simulink library "exampleMicrogridLibrary"  (R2020a)
settings: Solver=VariableStepAuto  StartTime=0.0  StopTime=10.0  RelTol=1e-3
undefined symbols (not defined in the file): BR, D1, Delta, DiscIntNeverNeededParam, Fnom, gcbh, Ion, kv, Lithium, Ls, Rs, sps_rtmsupport, StationData, Ts, Ts_Control, Vrms
libraries: powerlib x75, simulink x29, powerlib_meascontrol x26, sps_avr x5, spsDieselMotorModel x3, electricdrivelib x2, re_lib x1
(part 6 of 6)

== system exampleMicrogridLibrary/Grid-Connected Battery (Multi-mode EMT Model)/Inverter Control/Current Control/Current Regulator ==
  note: Current Regulator
      | ================
  note: Sign Convention: Current going out of the converter = positive current
  note: Iq positive --> The converter absorbs reactive power ("Inductive mode") = Reactive Power Q negative
  note: Id positive --> The converter generates active power ("Inverter mode") = Active Power P positive
  VdVq_meas : Inport  PortDimensions=2
  IdIq_meas : Inport  Port=2  PortDimensions=2
  IdIq_ref : Inport  Port=3  PortDimensions=2
  Add1 : Sum  Inputs=++-
  Add2 : Sum
  Add3 : Sum  Inputs=+++
  Demux : Demux  Outputs=2
  Demux1 : Demux  Outputs=2
  Lff : Gain  Gain=Ltot_pu  SaturateOnIntegerOverflow=on  OutDataTypeStr=Inherit: Same as input  ParamDataTypeStr=Inherit: Same as input
  "Lff  " : Gain  Gain=Ltot_pu  SaturateOnIntegerOverflow=on  OutDataTypeStr=Inherit: Same as input  ParamDataTypeStr=Inherit: Same as input
  Mux : Mux  Inputs=2
  PI : simulink/Continuous/PID Controller  Controller=PI  Form=Parallel  TimeDomain=Discrete-time  UseExternalTs=off  SampleTime=Ts_Control  IntegratorMethod=Forward Euler  FilterMethod=Forward Euler  ControllerParametersSource=internal  P=Kp_Ireg  I=Ki_Ireg  D=0  UseFilter=on  N=100  TunerSelectOption=Transfer Function Based (PID Tuner App)  InitialConditionSource=internal  InitialConditionForIntegrator=0  InitialConditionForFilter=0  DifferentiatorICPrevScaledInput=0  ExternalReset=none  TrackingMode=off  Kt=1  LimitOutput=on  UpperSaturationLimit=1.5  LowerSaturationLimit=-1.5  LinearizeAsGain=off  AntiWindupMode=clamping  Kb=1  POutMin=[]  POutMax=[]  IOutMin=[]  IOutMax=[]  DOutMin=[]  DOutMax=[]  NOutMin=[]  NOutMax=[]  SumOutMin=[]  SumOutMax=[]  SaturationOutMin=[]  SaturationOutMax=[]  PParamMin=[]  PParamMax=[]  IParamMin=[]  IParamMax=[]  DParamMin=[]  DParamMax=[]  NParamMin=[]  NParamMax=[]  KbParamMin=[]  KbParamMax=[]  KtParamMin=[]  KtParamMax=[]  KbOutMin=[]  KbOutMax=[]  KtOutMin=[]  KtOutMax=[]  IntegratorOutMin=[]  IntegratorOutMax=[]  FilterOutMin=[]  FilterOutMax=[]  SumI1OutMin=[]  SumI1OutMax=[]  SumI2OutMin=[]  SumI2OutMax=[]  SumI3OutMin=[]  SumI3OutMax=[]  SumI4OutMin=[]  SumI4OutMax=[]  SumDOutMin=[]  SumDOutMax=[]  DifferentiatorOutMin=[]  DifferentiatorOutMax=[]  FilterDiffOutCoefMin=[]  FilterDiffOutCoefMax=[]  ReciprocalOutMin=[]  ReciprocalOutMax=[]  SumDenOutMin=[]  SumDenOutMax=[]  SumNumOutMin=[]  SumNumOutMax=[]  DivideOutMin=[]  DivideOutMax=[]  UdiffTsProdOutMin=[]  UdiffTsProdOutMax=[]  NTsProdOutMin=[]  NTsProdOutMax=[]  UintegralTsProdOutMin=[]  UintegralTsProdOutMax=[]  UngainTsProdOutMin=[]  UngainTsProdOutMax=[]  IntegratorContinuousStateAttributes=''  IntegratorStateMustResolveToSignalObject=off  IntegratorRTWStateStorageClass=Auto  FilterContinuousStateAttributes=''  FilterStateMustResolveToSignalObject=off  FilterRTWStateStorageClass=Auto  ParallelPVariant=InternalParameters  IdealPVariant=Disabled  IVariant=InternalParameters  DVariant=Disabled  IntegratorVariant=Discrete  SatVariant=Enabled  AWVariant=DiscClampingParallel  PCopyVariant=Disabled  TRVariant=Disabled  FdbkBlocksVariant=Forward  IdealPFdbkVariant=Disabled  SatFdbkVariant=Disabled  DerivativeFilterVariant=Disabled  NVariant=Disabled  NCopyVariant=Disabled_SignalSpec  FilterICVariant=Disabled  IntegratorICVariant=InternalICs  ExternalResetVariant=Disabled  TRSumVariant=Passthrough  SumFdbkVariant=Disabled  SumVariant=Sum_PI  TsampFilterVariant=InternalTs  TsampNgainVariant=Passthrough  TsampIntegralVariant=Passthrough
  Rff : Gain  Gain=Rtot_pu  SaturateOnIntegerOverflow=on  OutDataTypeStr=Inherit: Same as input  ParamDataTypeStr=Inherit: Same as input
  "Rff " : Gain  Gain=Rtot_pu  SaturateOnIntegerOverflow=on  OutDataTypeStr=Inherit: Same as input  ParamDataTypeStr=Inherit: Same as input
  Saturation : Saturate  UpperLimit=1.5  LowerLimit=-1.5
  Scope : Scope  NumInputPorts=2
  Sum : Sum  Inputs=|-+
  VdVq_conv : Outport  VectorParamsAs1DForOutWhenUnconnected=off
  wires:
  Mux/1 -> Add2/2
  PI/1 -> Scope/2, Add2/1  "PI"
  Sum/1 -> Scope/1, PI/1
  IdIq_ref/1 -> Sum/2, Demux1/1
  IdIq_meas/1 -> Sum/1
  Add2/1 -> Saturation/1
  Saturation/1 -> VdVq_conv/1
  VdVq_meas/1 -> Demux/1
  Demux/1 -> Add1/1
  "Rff "/1 -> Add1/2
  Demux1/1 -> "Rff "/1, Lff/1
  "Lff  "/1 -> Add1/3
  Demux1/2 -> "Lff  "/1, Rff/1
  Rff/1 -> Add3/2
  Lff/1 -> Add3/3
  Add1/1 -> Mux/1  "Feedforward"
  Demux/2 -> Add3/1
  Add3/1 -> Mux/2

== system exampleMicrogridLibrary/Grid-Connected Battery (Multi-mode EMT Model)/Inverter Control/Current Control/Uabc_ref Generation max (m) = 1 ==
  note: (Correction for transformer
      |  D1 connection)
  note: (Correction for delai of Ts_Control)
  note: Uref Generation
      | ==============
  wt : Inport
  VdVq_conv : Inport  Port=2
  Add1 : Sum  Inputs=++++
  Add2 : Sum
  Complex to Magnitude-Angle : ComplexToMagnitudeAngle
  Constant : Constant  Value=-pi/6
  Constant1 : Constant  Value=Vnom_dc
  Constant2 : Constant  Value="[ 0  -2*pi/3  2*pi/3  ]"
  Constant3 : Constant  Value=Vnom_sec*sqrt(2)/sqrt(3)
  Constant4 : Constant  Value=Ts_Control*Fnom*(2*pi)
  Demux1 : Demux  Outputs=2
  Gain1 : Gain  Gain=1/2
  Product : Product  Inputs=*/  RndMeth=Zero
  Product1 : Product  Inputs=*/  RndMeth=Zero
  Product2 : Product  Inputs=**  RndMeth=Zero
  Real-Imag to Complex : RealImagToComplex
  Trigonometric Function : Trigonometry
  Uabc_ref : Outport  VectorParamsAs1DForOutWhenUnconnected=off
  wires:
  Constant1/1 -> Gain1/1
  VdVq_conv/1 -> Product1/1
  Product1/1 -> Demux1/1
  Gain1/1 -> Product/1
  Real-Imag to Complex/1 -> Complex to Magnitude-Angle/1
  Demux1/1 -> Real-Imag to Complex/1
  Demux1/2 -> Real-Imag to Complex/2
  Constant2/1 -> Add1/2
  Constant/1 -> Add1/3
  Constant3/1 -> Product/2
  Product/1 -> Product1/2
  Complex to Magnitude-Angle/2 -> Add2/1
  Add1/1 -> Add2/2
  Add2/1 -> Trigonometric Function/1
  Complex to Magnitude-Angle/1 -> Product2/1
  Trigonometric Function/1 -> Product2/2
  Product2/1 -> Uabc_ref/1
  wt/1 -> Add1/1
  Constant4/1 -> Add1/4

== system exampleMicrogridLibrary/Power Equation Wind Turbine (PQ Model)/Wind Turbine Power Equation/Wind Turbine Properties/Properties ==
  In1 : Inport
  Air Density : Gain  Gain=rho
  Blade Swept Area (m^2) : Gain  Gain=A
  Gain : Gain  Gain=1/2
  Power Coefficient : Constant  Value=Cp
  "Product " : Product  SaturateOnIntegerOverflow=on  OutDataTypeStr=Inherit: Same as first input
  wind_speed^3 : Fcn  Expr=u(1)^3
  Out1 : Outport  VectorParamsAs1DForOutWhenUnconnected=off
  wires:
  Blade Swept Area (m^2)/1 -> "Product "/1
  wind_speed^3/1 -> Air Density/1
  Power Coefficient/1 -> "Product "/2
  In1/1 -> wind_speed^3/1
  Air Density/1 -> Gain/1
  "Product "/1 -> Out1/1
  Gain/1 -> Blade Swept Area (m^2)/1

== system exampleMicrogridLibrary/Relay/Breaker (Pure Discrete)/Breaker A/Model ==
  "gate " : Inport
  Uswitch : Inport  Port=2
  C4 : Constant  Value=BR.com
  Data Type Conversion : DataTypeConversion  OutDataTypeStr=double  SaturateOnIntegerOverflow=on  RndMeth=Zero
  Switch3 : Switch  Threshold=0.5  ZeroCross=off  InputSameDT=on
  This signal is not used : Terminator
  Timer : Subsystem  DialogController=POWERSYS.PowerSysDialog  mask(Timer){t=BR.SwitchingTimes, e=BR.switchings}
      mask prompts: t "Time (s):"; e "Amplitude:"
      mask help:
      | Generates a signal changing at specified times.
      |
      | If a signal value is not specified at time zero, the output is kept at 0 until the first specified transition time.
      mask init: same as exampleMicrogridLibrary/Fault /Fault A/Model/Timer
      mask Help: helpview(psbhelp)
      mask Display: plot( tv(2:end-1), opv(2:end-1) )
  gate : Outport  VectorParamsAs1DForOutWhenUnconnected=off
  wires:
  Uswitch/1 -> This signal is not used/1
  C4/1 -> Switch3/2
  Timer/1(Out) -> Switch3/3
  Data Type Conversion/1 -> Switch3/1
  Switch3/1 -> gate/1
  "gate "/1 -> Data Type Conversion/1

== system exampleMicrogridLibrary/Relay/Breaker (Pure Discrete)/Breaker B/Model ==
  "gate " : Inport
  Uswitch : Inport  Port=2
  C4 : Constant  Value=BR.com
  Data Type Conversion : DataTypeConversion  OutDataTypeStr=double  SaturateOnIntegerOverflow=on  RndMeth=Zero
  Switch3 : Switch  Threshold=0.5  ZeroCross=off  InputSameDT=on
  This signal is not used : Terminator
  Timer : Subsystem  DialogController=POWERSYS.PowerSysDialog  mask(Timer){t=BR.SwitchingTimes, e=BR.switchings}
      mask prompts: t "Time (s):"; e "Amplitude:"
      mask help:
      | Generates a signal changing at specified times.
      |
      | If a signal value is not specified at time zero, the output is kept at 0 until the first specified transition time.
      mask init: same as exampleMicrogridLibrary/Fault /Fault A/Model/Timer
      mask Help: helpview(psbhelp)
      mask Display: plot( tv(2:end-1), opv(2:end-1) )
  gate : Outport  VectorParamsAs1DForOutWhenUnconnected=off
  wires:
  Uswitch/1 -> This signal is not used/1
  C4/1 -> Switch3/2
  Timer/1(Out) -> Switch3/3
  Data Type Conversion/1 -> Switch3/1
  Switch3/1 -> gate/1
  "gate "/1 -> Data Type Conversion/1

== system exampleMicrogridLibrary/Relay/Breaker (Pure Discrete)/Breaker C/Model ==
  "gate " : Inport
  Uswitch : Inport  Port=2
  C4 : Constant  Value=BR.com
  Data Type Conversion : DataTypeConversion  OutDataTypeStr=double  SaturateOnIntegerOverflow=on  RndMeth=Zero
  Switch3 : Switch  Threshold=0.5  ZeroCross=off  InputSameDT=on
  This signal is not used : Terminator
  Timer : Subsystem  DialogController=POWERSYS.PowerSysDialog  mask(Timer){t=BR.SwitchingTimes, e=BR.switchings}
      mask prompts: t "Time (s):"; e "Amplitude:"
      mask help:
      | Generates a signal changing at specified times.
      |
      | If a signal value is not specified at time zero, the output is kept at 0 until the first specified transition time.
      mask init: same as exampleMicrogridLibrary/Fault /Fault A/Model/Timer
      mask Help: helpview(psbhelp)
      mask Display: plot( tv(2:end-1), opv(2:end-1) )
  gate : Outport  VectorParamsAs1DForOutWhenUnconnected=off
  wires:
  Uswitch/1 -> This signal is not used/1
  C4/1 -> Switch3/2
  Timer/1(Out) -> Switch3/3
  Data Type Conversion/1 -> Switch3/1
  Switch3/1 -> gate/1
  "gate "/1 -> Data Type Conversion/1

== system exampleMicrogridLibrary/SPS-Simulink Interface/EMT/Frequency Generator/Continuous ==
  Clock : Clock
  Constant4 : Constant  Value=2*pi
  Freq1 : Constant  Value=Freq
  Freq2 : Constant  Value=2*pi
  Math Function : Math  Operator=mod  SignedPower=on  SaturateOnIntegerOverflow=on
  Product3 : Product  Inputs=***  InputSameDT=on  SaturateOnIntegerOverflow=on  OutDataTypeStr=Inherit: Same as first input
  2pi*f : Outport  VectorParamsAs1DForOutWhenUnconnected=off
  wires:
  Clock/1 -> Product3/2
  Freq2/1 -> Product3/3
  Freq1/1 -> Product3/1
  Constant4/1 -> Math Function/2
  Product3/1 -> Math Function/1
  Math Function/1 -> 2pi*f/1

== system exampleMicrogridLibrary/SPS-Simulink Interface/EMT/Frequency Generator/Discrete ==
  Constant4 : Constant  Value=2*pi
  Freq1 : Constant  Value=Freq
  Freq2 : Constant  Value=2*pi
  Math Function : Math  Operator=mod  SignedPower=on  SaturateOnIntegerOverflow=on
  Product3 : Product  Inputs=***  InputSameDT=on  SaturateOnIntegerOverflow=on  OutDataTypeStr=Inherit: Same as first input
  t : DigitalClock  SampleTime=Ts
  2pi*f : Outport  VectorParamsAs1DForOutWhenUnconnected=off
  wires:
  Math Function/1 -> 2pi*f/1
  Product3/1 -> Math Function/1
  Constant4/1 -> Math Function/2
  Freq1/1 -> Product3/1
  Freq2/1 -> Product3/3
  t/1 -> Product3/2

== system exampleMicrogridLibrary/Relay/Breaker (Pure Discrete)/Breaker A/Model/Timer ==
  Derivative : Derivative  Commented=on
  Digital Clock : DigitalClock  SampleTime=Ts
  Hit Crossing : HitCross  Commented=on  ShowOutputPort=off
  Look-Up Table : Lookup  InputValues=tv  Table=opv  SaturateOnIntegerOverflow=on
  Out : Outport  VectorParamsAs1DForOutWhenUnconnected=off
  wires:
  Derivative/1 -> Hit Crossing/1
  Look-Up Table/1 -> Derivative/1, Out/1
  Digital Clock/1 -> Look-Up Table/1

== system exampleMicrogridLibrary/Relay/Breaker (Pure Discrete)/Breaker B/Model/Timer ==
  Derivative : Derivative  Commented=on
  Digital Clock : DigitalClock  SampleTime=Ts
  Hit Crossing : HitCross  Commented=on  ShowOutputPort=off
  Look-Up Table : Lookup  InputValues=tv  Table=opv  SaturateOnIntegerOverflow=on
  Out : Outport  VectorParamsAs1DForOutWhenUnconnected=off
  wires:
  Derivative/1 -> Hit Crossing/1
  Look-Up Table/1 -> Derivative/1, Out/1
  Digital Clock/1 -> Look-Up Table/1

== system exampleMicrogridLibrary/Relay/Breaker (Pure Discrete)/Breaker C/Model/Timer ==
  Derivative : Derivative  Commented=on
  Digital Clock : DigitalClock  SampleTime=Ts
  Hit Crossing : HitCross  Commented=on  ShowOutputPort=off
  Look-Up Table : Lookup  InputValues=tv  Table=opv  SaturateOnIntegerOverflow=on
  Out : Outport  VectorParamsAs1DForOutWhenUnconnected=off
  wires:
  Derivative/1 -> Hit Crossing/1
  Look-Up Table/1 -> Derivative/1, Out/1
  Digital Clock/1 -> Look-Up Table/1

== matlab function exampleMicrogridLibrary/Solar Array (EMT Model)/Inverter Control/MPPT Controller using Perturbe & Observe technique  ==
  settings: updateMethod=DISCRETE  sampleTime=Ts_Control
  data: Param input; Enabled input; V input =V; I input; D output
function D  = PandO(Param, Enabled, V, I)

% MPPT controller based on the Perturb & Observe algorithm.

% D output = Reference for DC link voltage (Vdc_ref) 
%
% Enabled input = 1 to enable the MPPT controller
% V input = PV array terminal voltage (V)
% I input = PV array current (A)
%
% Param input:
Dinit = Param(1);  %Initial value for Vdc_ref
Dmax = Param(2);   %Maximum value for Vdc_ref
Dmin = Param(3);   %Minimum value for Vdc_ref
deltaD = Param(4); %Increment value used to increase/decrease Vdc_ref
%  

persistent Vold Pold Dold;

dataType = 'double';

if isempty(Vold)
    Vold=0;
    Pold=0;
    Dold=Dinit;
end
P= V*I;
dV= V - Vold;
dP= P - Pold;

if dP ~= 0 & Enabled ~=0
    if dP < 0
        if dV < 0
            D = Dold + deltaD;
        else
            D = Dold - deltaD;
        end
    else
        if dV < 0
            D = Dold - deltaD;
        else
            D = Dold + deltaD;
        end    
    end
else D=Dold;
end

if D >= Dmax | D<= Dmin
    D=Dold;
end

Dold=D;
Vold=V;
Pold=P;
